simulink model "high_pass_filter"  (R2020b)
settings: Solver=VariableStepAuto  StartTime=0.0  StopTime=10.0  RelTol=1e-3
settings Model: Creator=user  LastModifiedBy=user

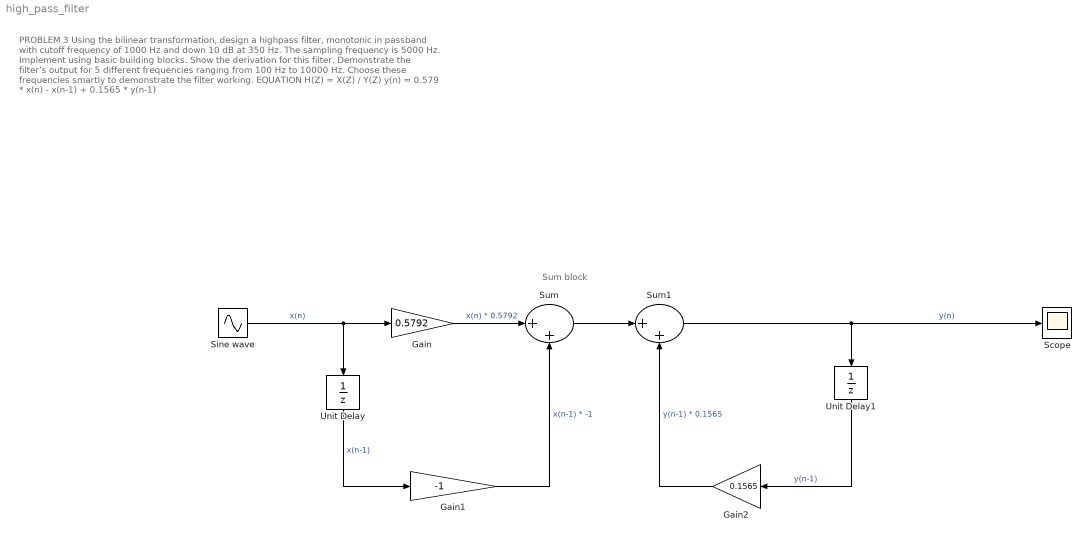
== system high_pass_filter ==
  note: Sum block
  note: PROBLEM 3
      |
      | Using the bilinear transformation, design a highpass filter, monotonic in passband with cutoff frequency of 1000 Hz and down 10 dB at 350 Hz. The sampling frequency is 5000 Hz. Implement using basic building blocks. Show the derivation for this filter. Demonstrate the filter’s output for 5 different frequencies ranging from 100 Hz to 10000 Hz. Choose these frequencies smartly to demonstrate the filter working.
      |
      | EQUATION
      | H(Z) = X(Z) / Y(Z)
      | y(n) = 0.579 * x(n) - x(n-1) + 0.1565 * y(n-1)
  Gain : Gain  Gain=0.5792
  Gain1 : Gain  Gain=-1
  Gain2 : Gain  Gain=0.1565
  Scope : Scope
  Sine wave : Sin  Frequency=7000*6.28  SampleTime=0
  Sum : Sum  Inputs=|++
  Sum1 : Sum  Inputs=|++
  Unit Delay : UnitDelay  SampleTime=-1  HasFrameUpgradeWarning=on
  Unit Delay1 : UnitDelay  SampleTime=-1  HasFrameUpgradeWarning=on
  wires:
  Sine wave/1 -> Unit Delay/1, Gain/1  "x(n)"
  Gain/1 -> Sum/1  "x(n) * 0.5792"
  Unit Delay/1 -> Gain1/1  "x(n-1)"
  Gain1/1 -> Sum/2  "x(n-1) * -1"
  Sum/1 -> Sum1/1
  Gain2/1 -> Sum1/2  "y(n-1) * 0.1565"
  Sum1/1 -> Unit Delay1/1, Scope/1  "y(n)"
  Unit Delay1/1 -> Gain2/1  "y(n-1)"
